simulink model "t5_2_Dinamica_Proyectil_Friccion"  (R2024a)
settings: Solver=FixedStepAuto  StartTime=0.0  StopTime=7  FixedStep=.01  RelTol=1e-3
StopFcn:
  | %data = [out.tout,out.x,out.y];
  | %save('EmpriricalData.mat','data')
model workspace (MATLAB code in the model file):
  | rho=0.074;
  | Cd=0.87;
  | A=0.2;
  | 
  | v0 = 30; %m/s
  | theta0 = pi/6;
settings Model: Creator=scpmoxxa  LastModifiedBy=pablo
settings OptimizationCC: ReuseModelBlockBuffer=off
settings DebuggingCC: UnconnectedInputMsg=warning  UnconnectedOutputMsg=warning  UnconnectedLineMsg=warning
settings ModelReferenceCC: EnableRefExpFcnMdlSchedulingChecks=on
settings RTWCC: GPUComputeCapability=3.5  DLArmComputeVersion=19.05

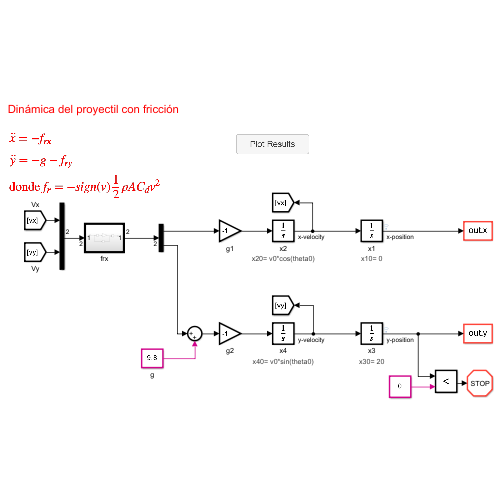
[thumbnail: Simulink's stored preview of the top-level diagram]
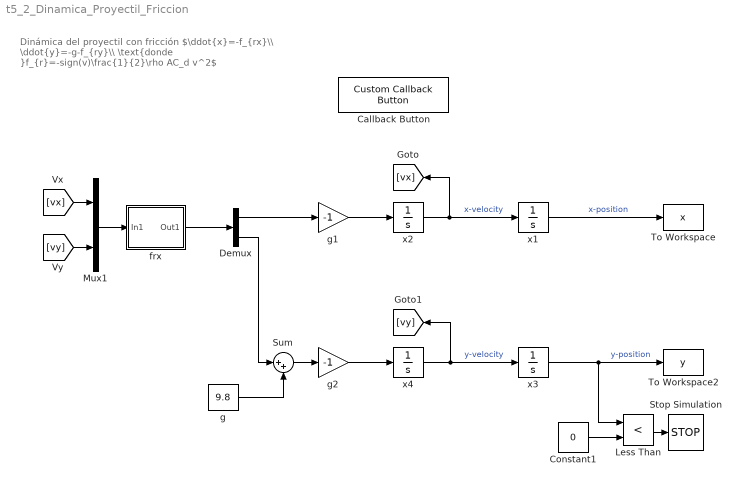
== system t5_2_Dinamica_Proyectil_Friccion ==
  note: Dinámica del proyectil con fricción
      |
      | $\ddot{x}=-f_{rx}\\ \ddot{y}=-g-f_{ry}\\ \text{donde }f_{r}=-sign(v)\frac{1}{2}\rho AC_d v^2$
  Callback Button : CustomCallbackButton  Configuration="{\"components\":[{\"name\":\"BackgroundImageComponent\",\"settings\":{\"image\":{\"size\":[0,0],\"src\":\"default\",\"srcOrientation\":\"Right\"},\"position\":[0,0,1,1]}},{\"name\":\"ButtonStateComponent\",\"settings\":{\"buttonType\":\"momentary\",\"clickFcn\":\"close all\\n\\nfigure;\\nplot(out.x,out.y)\\nxlabel('x');ylabel('y')\\n\\n\",\"onValue\":1,\"position\":[0,0,1,1],\"pressDelay\":\"500\",\"pressFcn\":\"\",\"repeatInterval\":\"0\",\"states\":[{\"horizontalAlignment\":\"center\",\"image\":{\"position\":[0,0,1,1],\"src\":\"default\",\"srcOrientation\":\"Right\"},\"label\":{\"color\":[0.01176470588,0.01176470588,0.01176470588,1],\"icon\":{\"size\":[0,0],\"src\":\"default\",\"srcOrientation\":\"Right\"},\"iconPlacement\":\"left\",\"text\":{\"content\":\"Plot Results\"}},\"labelOffset\":[0,0],\"verticalAlignment\":\"middle\"},{\"horizontalAlignment\":\"center\",\"image\":{\"position\":[0,0,1,1],\"src\":\"default\",\"srcOrientation\":\"Right\"},\"label\":{\"color\":[0.01176470588,0.01176470588,0.01176470588,1],\"icon\":{\"size\":[0,0],\"src\":\"default\",\"srcOrientation\":\"Right\"},\"iconPlacement\":\"left\",\"text\":{\"content\":\"Plot Results\"}},\"labelOffset\":[0,0],\"verticalAlignment\":\"middle\"},{\"horizontalAlignment\":\"center\",\"image\":{\"position\":[0,0,1,1],\"src\":\"default\",\"srcOrientation\":\"Right\"},\"label\":{\"color\":[0.01176470588,0.01176470588,0.01176470588,1],\"icon\":{\"size\":[0,0],\"src\":\"default\",\"srcOrientation\":\"Right\"},\"iconPlacement\":\"left\",\"text\":{\"content\":\"Plot Results\"}},\"labelOffset\":[0,0],\"verticalAlignment\":\"middle\"},{\"horizontalAlignment\":\"center\",\"image\":{\"position\":[0,0,1,1],\"src\":\"default\",\"srcOrientation\":\"Right\"},\"label\":{\"color\":[0.01176470588,0.01176470588,0.01176470588,1],\"icon\":{\"size\":[0,0],\"src\":\"default\",\"srcOrientation\":\"Right\"},\"iconPlacement\":\"left\",\"text\":{\"content\":\"Plot Results\"}},\"labelOffset\":[0,0],\"verticalAlignment\":\"middle\"}]}},{\"name\":\"ForegroundImageComponent\",\"settings\":{\"image\":{\"size\":[0,0],\"src\":\"default\",\"srcOrientation\":\"Right\"},\"isForeground\":1,\"position\":[0,0,1,1]}}],\"settings\":{\"BindingType\":\"standalone\",\"backgroundColor\":[244,244,244,1],\"backgroundOffset\":0.2,\"backgroundOpacity\":1,\"fixedAspectRatio\":\"off\",\"foregroundColor\":[0.01176470588,0.01176470588,0.01176470588,1],\"migratedFromLegacy\":true,\"useBackgroundColor\":true,\"variant\":\"callback\",\"version\":\"R2023a\"},\"type\":\"Button\"}"  CustomBackgroundColor="{\"color\":[0.9568627451,0.9568627451,0.9568627451],\"show\":true}"
  Constant1 : Constant  Value=0
  Demux : Demux  Outputs=2
  Less Than : RelationalOperator  Operator=<  OutDataTypeStr=boolean  RndMeth=Simplest  InputSameDT=off
  Mux1 : Mux  Inputs=2
  Stop Simulation : Stop
  Sum : Sum  Inputs=|++
  To Workspace : ToWorkspace  VariableName=x  SampleTime=-1
  To Workspace2 : ToWorkspace  VariableName=y  SampleTime=-1
  frx : Subsystem  TreatAsAtomicUnit=on
  g : Constant  Value=9.8
  g1 : Gain  Gain=-1
  g2 : Gain  Gain=-1
  x1 : Integrator
      settings: AttributesFormatString=x10= %<InitialCondition>
  x2 : Integrator  InitialCondition=v0*cos(theta0)
      settings: AttributesFormatString=x20= %<InitialCondition>
  x3 : Integrator  InitialCondition=20
      settings: AttributesFormatString=x30= %<InitialCondition>
  x4 : Integrator  InitialCondition=v0*sin(theta0)
      settings: AttributesFormatString=x40= %<InitialCondition>
  wires:
  x2/1 -> [vx], x1/1  "x-velocity"
  g/1 -> Sum/2
  g1/1 -> x2/1
  g2/1 -> x4/1
  x4/1 -> [vy], x3/1  "y-velocity"
  Sum/1 -> g2/1
  frx/1(Out1) -> Demux/1
  Demux/1 -> g1/1
  Demux/2 -> Sum/1
  Mux1/1 -> frx/1(In1)
  Constant1/1 -> Less Than/2
  Less Than/1 -> Stop Simulation/1
  x1/1 -> To Workspace/1  "x-position"
  x3/1 -> Less Than/1, To Workspace2/1  "y-position"
  [vx] -> Mux1/1
  [vy] -> Mux1/2

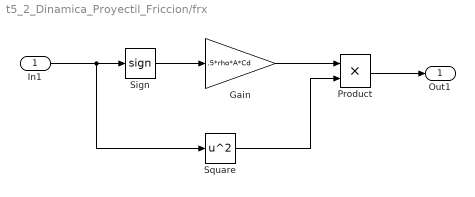
== system t5_2_Dinamica_Proyectil_Friccion/frx ==
  In1 : Inport
  Gain : Gain  Gain=.5*rho*A*Cd
  Product : Product
  Sign : Signum
  Square : Math  Operator=square
  Out1 : Outport
  wires:
  Square/1 -> Product/2
  In1/1 -> Square/1, Sign/1
  Gain/1 -> Product/1
  Product/1 -> Out1/1
  Sign/1 -> Gain/1
